simulink model "H333_LOEKnown_400HzMIL"  (R2020b)
settings: Solver=ode4  StartTime=0.0  StopTime=60  FixedStep=Ts  RelTol=1e-3
undefined symbols (not defined in the file): DiscIntNeverNeededParam, Ts
libraries: sharedtransform x3, dspnetwork x1
settings Model: EnablePacing=on  Creator=kcx06  LastModifiedBy=kcx06

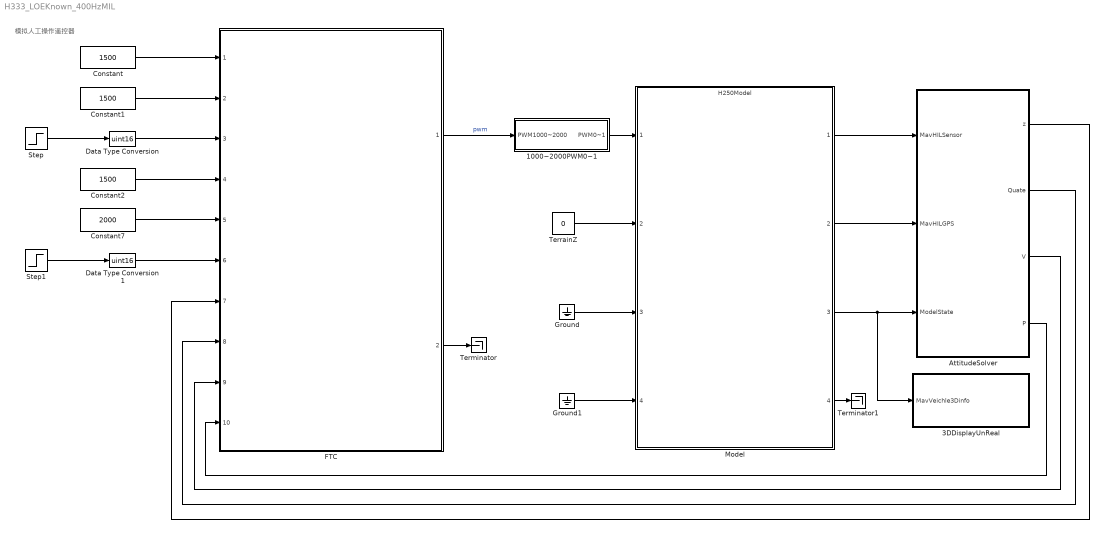
== system H333_LOEKnown_400HzMIL ==
  note: 模拟人工操作遥控器
  1000~2000PWM0~1 : Subsystem
  3DDisplayUnReal : Subsystem
  AttitudeSolver : Subsystem
  Constant : Constant  Value=1500  OutDataTypeStr=uint16  SampleTime=Ts
  Constant1 : Constant  Value=1500  OutDataTypeStr=uint16  SampleTime=Ts
  Constant2 : Constant  Value=1500  OutDataTypeStr=uint16
  Constant7 : Constant  Value=2000  OutDataTypeStr=uint16
  Data Type Conversion : DataTypeConversion  OutDataTypeStr=uint16
  Data Type Conversion1 : DataTypeConversion  OutDataTypeStr=uint16
  FTC : Subsystem  ReferencedSubsystem=FTC
  Ground : Ground
  Ground1 : Ground
  Model : ModelReference  ModelNameDialog=H250Model.slx  SimulationMode=Normal  ModelReferenceVersion=2.31
  Step : Step  Time=10  Before=1900  After=1500  OutDataTypeStr=single  SampleTime=Ts
  Step1 : Step  Time=15  Before=1000  After=2000  OutDataTypeStr=single  SampleTime=Ts
  Terminator : Terminator
  Terminator1 : Terminator
  TerrainZ : Constant  Value=0
  wires:
  Model/3 -> AttitudeSolver/3(ModelState), 3DDisplayUnReal/1(MavVeichle3Dinfo)
  FTC/1 -> 1000~2000PWM0~1/1(PWM1000~2000)  "pwm"
  1000~2000PWM0~1/1(PWM0~1) -> Model/1
  FTC/2 -> Terminator/1
  TerrainZ/1 -> Model/2
  Model/1 -> AttitudeSolver/1(MavHILSensor)
  Model/2 -> AttitudeSolver/2(MavHILGPS)
  AttitudeSolver/1(z) -> FTC/7
  AttitudeSolver/2(Quate) -> FTC/8
  AttitudeSolver/3(V) -> FTC/9
  AttitudeSolver/4(P) -> FTC/10
  Constant/1 -> FTC/1
  Constant2/1 -> FTC/4
  Step/1 -> Data Type Conversion/1
  Constant7/1 -> FTC/5
  Data Type Conversion/1 -> FTC/3
  Step1/1 -> Data Type Conversion1/1
  Data Type Conversion1/1 -> FTC/6
  Model/4 -> Terminator1/1
  Ground/1 -> Model/3
  Ground1/1 -> Model/4
  Constant1/1 -> FTC/2

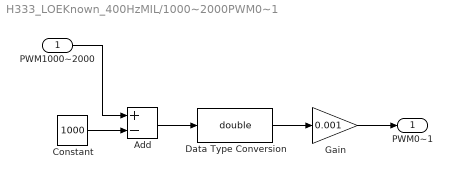
== system H333_LOEKnown_400HzMIL/1000~2000PWM0~1 ==
  PWM1000~2000 : Inport
  Add : Sum  Inputs=+-
  Constant : Constant  Value=1000
  Data Type Conversion : DataTypeConversion  OutDataTypeStr=double
  Gain : Gain  Gain=0.001
  PWM0~1 : Outport
  wires:
  PWM1000~2000/1 -> Add/1
  Constant/1 -> Add/2
  Gain/1 -> PWM0~1/1
  Data Type Conversion/1 -> Gain/1
  Add/1 -> Data Type Conversion/1

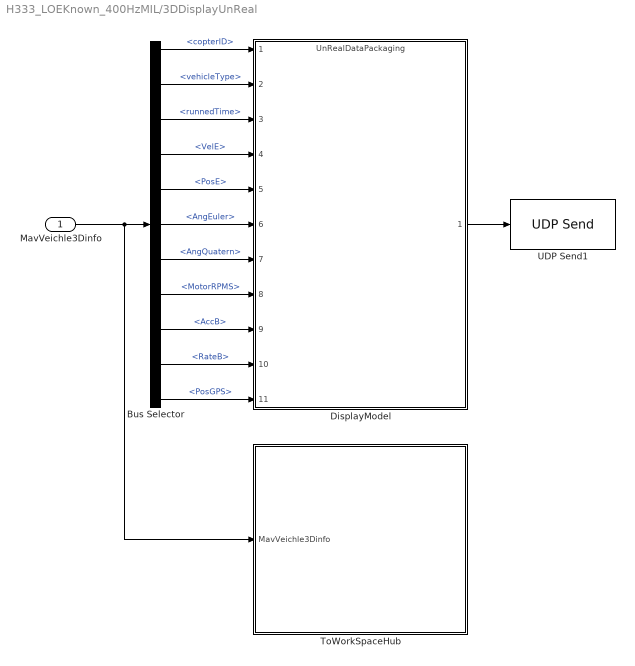
== system H333_LOEKnown_400HzMIL/3DDisplayUnReal ==
  MavVeichle3Dinfo : Inport
  Bus Selector : BusSelector  OutputSignals=copterID,vehicleType,runnedTime,VelE,PosE,AngEuler,AngQuatern,MotorRPMS,AccB,RateB,PosGPS
  DisplayModel : ModelReference  ModelNameDialog=UnRealDataPackaging.slx  ModelReferenceVersion=1.123
  ToWorkSpaceHub : Subsystem
  UDP Send1 : dspnetwork/UDP Send  remoteURL='127.0.0.1'  remotePort=20010  localURL='0.0.0.0'  localPortSource=Automatically determine  localPort=20011  sendBufferSize=8192  sampletime=-1  blockPlatform=[]  separateLengthPort=0
  wires:
  Bus Selector/10 -> DisplayModel/10  "<RateB>"
  Bus Selector/2 -> DisplayModel/2  "<vehicleType>"
  MavVeichle3Dinfo/1 -> ToWorkSpaceHub/1(MavVeichle3Dinfo), Bus Selector/1
  Bus Selector/8 -> DisplayModel/8  "<MotorRPMS>"
  Bus Selector/7 -> DisplayModel/7  "<AngQuatern>"
  Bus Selector/1 -> DisplayModel/1  "<copterID>"
  Bus Selector/6 -> DisplayModel/6  "<AngEuler>"
  Bus Selector/9 -> DisplayModel/9  "<AccB>"
  Bus Selector/5 -> DisplayModel/5  "<PosE>"
  Bus Selector/11 -> DisplayModel/11  "<PosGPS>"
  Bus Selector/3 -> DisplayModel/3  "<runnedTime>"
  Bus Selector/4 -> DisplayModel/4  "<VelE>"
  DisplayModel/1 -> UDP Send1/1

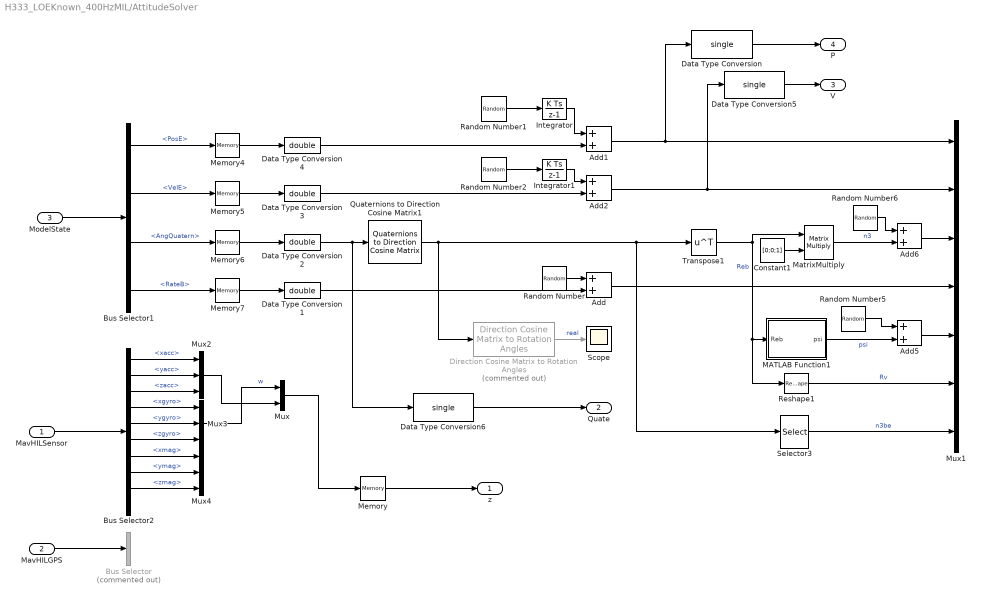
== system H333_LOEKnown_400HzMIL/AttitudeSolver ==
  MavHILSensor : Inport
  MavHILGPS : Inport  Port=2
  ModelState : Inport  Port=3
  Add{,1..2,5..6} (5 alike) : Sum
  Bus Selector : BusSelector  Commented=on  OutputSignals=lat,lon,alt,vn,ve,vd  OutputAsBus=on
  Bus Selector1 : BusSelector  OutputSignals=PosE,VelE,AngQuatern,RateB
  Bus Selector2 : BusSelector  OutputSignals=xacc,yacc,zacc,xgyro,ygyro,zgyro,xmag,ymag,zmag,pressure_alt
  Constant1 : Constant  Value=[0;0;1]
  Data Type Conversion : DataTypeConversion  OutDataTypeStr=single
  Data Type Conversion{1..4} (4 alike) : DataTypeConversion  OutDataTypeStr=double
  Data Type Conversion5 : DataTypeConversion  OutDataTypeStr=single
  Data Type Conversion6 : DataTypeConversion  OutDataTypeStr=single
  Direction Cosine Matrix to Rotation Angles : sharedtransform/Direction Cosine Matrix to Rotation Angles  Commented=on  rotationOrder=ZYX  aMode=aMode  action=None  tolerance=eps(2)
      settings: SourceProductBaseCode=AE,PW,MT,UV,VE,VP
  Integrator : DiscreteIntegrator  SampleTime=Ts  ICPrevOutput=DiscIntNeverNeededParam  ICPrevScaledInput=DiscIntNeverNeededParam  mask(DiscretizedDiscreteIntegrator){}
      mask init:
      | %zoh
  Integrator1 : DiscreteIntegrator  SampleTime=Ts  ICPrevOutput=DiscIntNeverNeededParam  ICPrevScaledInput=DiscIntNeverNeededParam  mask(DiscretizedDiscreteIntegrator){}
      mask init:
      | %zoh
  MATLAB Function1 : MATLAB Function  TreatAsAtomicUnit=on
  MatrixMultiply : Product  Multiplication=Matrix(*)
  Memory : Memory
  Memory4 : Memory  InitialCondition=[0;0;0]
  Memory5 : Memory  InitialCondition=[0;0;0]
  Memory6 : Memory  InitialCondition=[1; 0; 0; 0]
  Memory7 : Memory  InitialCondition=[0;0;0]
  Mux : Mux  Inputs=2
  Mux1 : Mux  Inputs=[3 3 3 3 1 9 3]
  Mux2 : Mux  Inputs=3
  Mux3 : Mux  Inputs=3
  Mux4 : Mux  Inputs=3
  Quaternions to Direction Cosine Matrix1 : sharedtransform/Quaternions to  Direction Cosine Matrix  aMode=aMode
      settings: SourceProductBaseCode=AE,PW,MT,UV,VE,VP
  Random Number : RandomNumber  Variance=0.001  Seed=[123 321 564]  SampleTime=Ts
  Random Number1 : RandomNumber  Variance=0.1  Seed=[10 20 15]  SampleTime=Ts
  Random Number2 : RandomNumber  Variance=0.1  Seed=[25 30 35]  SampleTime=Ts
  Random Number5 : RandomNumber  Variance=0.00002  Seed=[12]  SampleTime=Ts*4
  Random Number6 : RandomNumber  Variance=0.00002  Seed=[98 99 100]  SampleTime=Ts*4
  Reshape1 : Reshape
  Scope : Scope
  Selector3 : Selector  NumberOfDimensions=2  InputPortWidth=3  IndexOptions=Select all,Index vector (dialog)  Indices=[1 3],3  OutputSizes=1,1
  Transpose1 : Math  Operator=transpose  SaturateOnIntegerOverflow=on
  z : Outport
  Quate : Outport  Port=2
  V : Outport  Port=3
  P : Outport  Port=4
  wires:
  Random Number/1 -> Add/1
  Integrator/1 -> Add1/1
  Random Number1/1 -> Integrator/1
  Random Number2/1 -> Integrator1/1
  Integrator1/1 -> Add2/1
  MavHILSensor/1 -> Bus Selector2/1
  Quaternions to Direction Cosine Matrix1/1 -> Direction Cosine Matrix to Rotation Angles/1, Selector3/1, Transpose1/1
  Bus Selector1/4 -> Memory7/1  "<RateB>"
  Add/1 -> Mux1/4
  Add2/1 -> Mux1/2, Data Type Conversion5/1
  Add1/1 -> Mux1/1, Data Type Conversion/1
  Add6/1 -> Mux1/3
  Transpose1/1 -> MatrixMultiply/1, MATLAB Function1/1(Reb), Reshape1/1  "Reb"
  Add5/1 -> Mux1/5
  Reshape1/1 -> Mux1/6  "Rv"
  MATLAB Function1/1(psi) -> Add5/2  "psi"
  MatrixMultiply/1 -> Add6/2  "n3"
  Random Number5/1 -> Add5/1
  Random Number6/1 -> Add6/1
  Selector3/1 -> Mux1/7  "n3be"
  Direction Cosine Matrix to Rotation Angles/1 -> Scope/1  "real"
  ModelState/1 -> Bus Selector1/1
  Bus Selector1/1 -> Memory4/1  "<PosE>"
  Bus Selector1/2 -> Memory5/1  "<VelE>"
  Bus Selector1/3 -> Memory6/1  "<AngQuatern>"
  MavHILGPS/1 -> Bus Selector/1
  Bus Selector2/1 -> Mux2/1  "<xacc>"
  Bus Selector2/2 -> Mux2/2  "<yacc>"
  Bus Selector2/3 -> Mux2/3  "<zacc>"
  Bus Selector2/5 -> Mux3/2  "<ygyro>"
  Bus Selector2/6 -> Mux3/3  "<zgyro>"
  Bus Selector2/4 -> Mux3/1  "<xgyro>"
  Bus Selector2/9 -> Mux4/3  "<zmag>"
  Bus Selector2/8 -> Mux4/2  "<ymag>"
  Bus Selector2/7 -> Mux4/1  "<xmag>"
  Data Type Conversion1/1 -> Add/2
  Data Type Conversion3/1 -> Add2/2
  Data Type Conversion4/1 -> Add1/2
  Memory4/1 -> Data Type Conversion4/1
  Memory5/1 -> Data Type Conversion3/1
  Memory6/1 -> Data Type Conversion2/1
  Memory7/1 -> Data Type Conversion1/1
  Constant1/1 -> MatrixMultiply/2
  Mux3/1 -> Mux/1  "w"
  Mux2/1 -> Mux/2
  Mux/1 -> Memory/1
  Data Type Conversion2/1 -> Data Type Conversion6/1, Quaternions to Direction Cosine Matrix1/1
  Data Type Conversion/1 -> P/1
  Data Type Conversion5/1 -> V/1
  Data Type Conversion6/1 -> Quate/1
  Memory/1 -> z/1

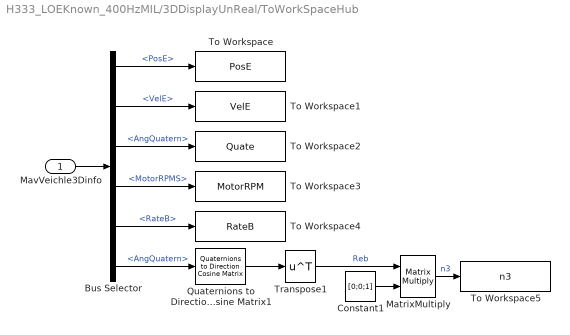
== system H333_LOEKnown_400HzMIL/3DDisplayUnReal/ToWorkSpaceHub ==
  MavVeichle3Dinfo : Inport
  Bus Selector : BusSelector  OutputSignals=PosE,VelE,AngQuatern,MotorRPMS,RateB,AngQuatern
  Constant1 : Constant  Value=[0;0;1]
  MatrixMultiply : Product  Multiplication=Matrix(*)
  Quaternions to Direction Cosine Matrix1 : sharedtransform/Quaternions to  Direction Cosine Matrix  aMode=aMode
      settings: SourceProductBaseCode=AE,PW,MT,UV,VE,VP
  To Workspace : ToWorkspace  VariableName=PosE  SaveFormat=Timeseries  SampleTime=-1
  To Workspace1 : ToWorkspace  VariableName=VelE  SaveFormat=Timeseries  SampleTime=-1
  To Workspace2 : ToWorkspace  VariableName=Quate  SaveFormat=Timeseries  SampleTime=-1
  To Workspace3 : ToWorkspace  VariableName=MotorRPM  SaveFormat=Timeseries  SampleTime=-1
  To Workspace4 : ToWorkspace  VariableName=RateB  SaveFormat=Timeseries  SampleTime=-1
  To Workspace5 : ToWorkspace  VariableName=n3  SaveFormat=Timeseries  SampleTime=-1
  Transpose1 : Math  Operator=transpose  SaturateOnIntegerOverflow=on
  wires:
  MavVeichle3Dinfo/1 -> Bus Selector/1
  Bus Selector/1 -> To Workspace/1  "<PosE>"
  Bus Selector/2 -> To Workspace1/1  "<VelE>"
  Bus Selector/3 -> To Workspace2/1  "<AngQuatern>"
  Bus Selector/4 -> To Workspace3/1  "<MotorRPMS>"
  Bus Selector/5 -> To Workspace4/1  "<RateB>"
  Constant1/1 -> MatrixMultiply/2
  Quaternions to Direction Cosine Matrix1/1 -> Transpose1/1
  Bus Selector/6 -> Quaternions to Direction Cosine Matrix1/1  "<AngQuatern>"
  Transpose1/1 -> MatrixMultiply/1  "Reb"
  MatrixMultiply/1 -> To Workspace5/1  "n3"

== matlab function H333_LOEKnown_400HzMIL/AttitudeSolver/MATLAB Function1 ==
  data: Reb input; psi output
function psi = fcn(Reb)
psi = atan2(Reb(2,1), Reb(1,1));
